simulink model "FSAC2021_V1_Running"  (R2014a)
settings: Solver=FixedStepDiscrete  StartTime=0.0  StopTime=inf  FixedStep=0.0005  RelTol=1e-3
model workspace (MAT data in the model file):
  MCOS : class17 (value not decoded)
  MCOS : class17 (value not decoded)
  MCOS : class17 (value not decoded)
  MCOS : class17 (value not decoded)
  MCOS : class17 (value not decoded)
  MCOS : class17 (value not decoded)
  MCOS : class17 (value not decoded)
  MCOS : class17 (value not decoded)
  MCOS : class17 (value not decoded)
  MCOS : class17 (value not decoded)
  MCOS : class17 (value not decoded)
  MCOS : class17 (value not decoded)
  MCOS : class17 (value not decoded)
  MCOS : class17 (value not decoded)
  MCOS : class17 (value not decoded)
  MCOS : class17 (value not decoded)
  MCOS : class17 (value not decoded)
  MCOS : class17 (value not decoded)
  MCOS : class17 (value not decoded)
  BUZZER_START = 1
  MCOS : class17 (value not decoded)
  MCOS : class17 (value not decoded)
  MCOS : class17 (value not decoded)
  MCOS : class17 (value not decoded)
  MCOS : class17 (value not decoded)
  MCOS : class17 (value not decoded)
  MCOS : class17 (value not decoded)
  MCOS : class17 (value not decoded)
  MCOS : class17 (value not decoded)
  MCOS : class17 (value not decoded)
  MCOS : class17 (value not decoded)
  MCOS : class17 (value not decoded)
  MCOS : class17 (value not decoded)
  MCOS : class17 (value not decoded)
  MCOS : class17 (value not decoded)
  MCOS : class17 (value not decoded)
  MCOS : class17 (value not decoded)
  MCOS : class17 (value not decoded)
  MCOS : class17 (value not decoded)
  MCOS : class17 (value not decoded)
  MCOS : class17 (value not decoded)
  MCOS : class17 (value not decoded)
  MCOS : class17 (value not decoded)
  MCOS : class17 (value not decoded)
  MCOS : class17 (value not decoded)
  MCOS : class17 (value not decoded)
  MCOS : class17 (value not decoded)
  MCOS : class17 (value not decoded)
  MCOS : class17 (value not decoded)
  MCOS : class17 (value not decoded)
  MCOS : class17 (value not decoded)
  MCOS : class17 (value not decoded)
  MCOS : class17 (value not decoded)
  MCOS : class17 (value not decoded)
  MCOS : class17 (value not decoded)
  MCOS : class17 (value not decoded)
  MCOS : class17 (value not decoded)
  MCOS : class17 (value not decoded)
  Brake = 11
  MCOS : class17 (value not decoded)
  MCOS : class17 (value not decoded)
  MCOS : class17 (value not decoded)
  MCOS : class17 (value not decoded)
  MCOS : class17 (value not decoded)
  MCOS : class17 (value not decoded)
  MCOS : class17 (value not decoded)
  MCOS : class17 (value not decoded)
  Sensor_Acc_b = 101.85
  Sensor_Acc_k = -0.0185
  Str_Sen_Orig_Angle = -341
  MCOS : class17 (value not decoded)
  Tire_D = 0.47
  T = 0.05
libraries: simulink x402, ec55xxlib x134
(part 17 of 17)

== system FSAC2021_V1_Running/ROUTING/TO_DCAN/Subsystem/DIAG_VEH_SENSOR/Front_wheel_angle ==
  Front_wheel_angle : Inport
  Constant{1..3,5..8} (7 alike) : Constant  Value=0  OutDataTypeStr=uint8  SampleTime=-1
  Front_wheel_angleABS : Abs
  Front_wheel_angleCS : ArithShift  BitShiftNumber=-8
  Front_wheel_angleConS : Constant  OutDataTypeStr=single
  Front_wheel_angleCosR : Constant  Value=0  OutDataTypeStr=uint8
  Front_wheel_angleROP : RelationalOperator  Operator=<  OutDataTypeStr=boolean
  Front_wheel_angleRon : Rounding  Operator=round
  Front_wheel_angleSW : Switch  Criteria=u2 ~= 0
  Front_wheel_angle_1sat : Saturate  UpperLimit=255  LowerLimit=0
  Front_wheel_angle_Convert : DataTypeConversion  OutDataTypeStr=uint8
  Front_wheel_angle_Convert1 : DataTypeConversion  OutDataTypeStr=uint32
  Front_wheel_angle_D : Product  Inputs=*/
  Front_wheel_angle_F : Constant  OutDataTypeStr=single
  Front_wheel_angle_L : simulink/Logic and Bit Operations/Bitwise Operator  logicop=AND  UseBitMask=on  BitMask=255  BitMaskRealWorld=Stored Integer
  Front_wheel_angle_O : Constant  Value=0  OutDataTypeStr=single
  Front_wheel_angle_S : ArithShift
  Front_wheel_angle_sat : Saturate  UpperLimit=127  LowerLimit=-128
  Front_wheel_angle_st : Sum  Inputs=+-
  Front_wheel_anglesubcon : Sum  Inputs=+-
  output1 : Outport
  output2 : Outport  Port=2
  output3 : Outport  Port=3
  output4 : Outport  Port=4
  output5 : Outport  Port=5
  output6 : Outport  Port=6
  output7 : Outport  Port=7
  output8 : Outport  Port=8
  wires:
  Front_wheel_angle/1 -> Front_wheel_angle_sat/1
  Front_wheel_angle_sat/1 -> Front_wheel_angle_st/1
  Front_wheel_angle_O/1 -> Front_wheel_angle_st/2
  Front_wheel_angle_st/1 -> Front_wheel_angle_D/1
  Front_wheel_angle_F/1 -> Front_wheel_angle_D/2
  Front_wheel_angle_D/1 -> Front_wheel_angleRon/1
  Front_wheel_angleRon/1 -> Front_wheel_angleROP/1, Front_wheel_angleABS/1, Front_wheel_angleSW/3
  Front_wheel_angleCosR/1 -> Front_wheel_angleROP/2
  Front_wheel_angleConS/1 -> Front_wheel_angleCS/1
  Front_wheel_angleCS/1 -> Front_wheel_anglesubcon/1
  Front_wheel_angleABS/1 -> Front_wheel_anglesubcon/2
  Front_wheel_anglesubcon/1 -> Front_wheel_angleSW/1
  Front_wheel_angleROP/1 -> Front_wheel_angleSW/2
  Front_wheel_angleSW/1 -> Front_wheel_angle_S/1
  Front_wheel_angle_S/1 -> Front_wheel_angle_1sat/1
  Front_wheel_angle_1sat/1 -> Front_wheel_angle_Convert1/1
  Front_wheel_angle_Convert1/1 -> Front_wheel_angle_L/1
  Front_wheel_angle_L/1 -> Front_wheel_angle_Convert/1
  Front_wheel_angle_Convert/1 -> output4/1
  Constant1/1 -> output1/1
  Constant2/1 -> output2/1
  Constant3/1 -> output3/1
  Constant5/1 -> output5/1
  Constant6/1 -> output6/1
  Constant7/1 -> output7/1
  Constant8/1 -> output8/1

== system FSAC2021_V1_Running/ROUTING/TO_DCAN/Subsystem/DIAG_VEH_SENSOR/Hydra_Prs ==
  Hydra_Prs : Inport
  Constant{1..4,6..8} (7 alike) : Constant  Value=0  OutDataTypeStr=uint8  SampleTime=-1
  Hydra_PrsRon : Rounding  Operator=round
  Hydra_Prs_1sat : Saturate  UpperLimit=255  LowerLimit=0
  Hydra_Prs_Convert : DataTypeConversion  OutDataTypeStr=uint8
  Hydra_Prs_Convert1 : DataTypeConversion  OutDataTypeStr=uint32
  Hydra_Prs_D : Product  Inputs=*/
  Hydra_Prs_F : Constant  Value=0.1  OutDataTypeStr=single
  Hydra_Prs_L : simulink/Logic and Bit Operations/Bitwise Operator  logicop=AND  UseBitMask=on  BitMask=255  BitMaskRealWorld=Stored Integer
  Hydra_Prs_O : Constant  Value=0  OutDataTypeStr=single
  Hydra_Prs_S : ArithShift
  Hydra_Prs_sat : Saturate  UpperLimit=25.5  LowerLimit=0
  Hydra_Prs_st : Sum  Inputs=+-
  output1 : Outport
  output2 : Outport  Port=2
  output3 : Outport  Port=3
  output4 : Outport  Port=4
  output5 : Outport  Port=5
  output6 : Outport  Port=6
  output7 : Outport  Port=7
  output8 : Outport  Port=8
  wires:
  Hydra_Prs/1 -> Hydra_Prs_sat/1
  Hydra_Prs_sat/1 -> Hydra_Prs_st/1
  Hydra_Prs_O/1 -> Hydra_Prs_st/2
  Hydra_Prs_st/1 -> Hydra_Prs_D/1
  Hydra_Prs_F/1 -> Hydra_Prs_D/2
  Hydra_Prs_D/1 -> Hydra_PrsRon/1
  Hydra_PrsRon/1 -> Hydra_Prs_S/1
  Hydra_Prs_S/1 -> Hydra_Prs_1sat/1
  Hydra_Prs_1sat/1 -> Hydra_Prs_Convert1/1
  Hydra_Prs_Convert1/1 -> Hydra_Prs_L/1
  Hydra_Prs_L/1 -> Hydra_Prs_Convert/1
  Hydra_Prs_Convert/1 -> output5/1
  Constant1/1 -> output1/1
  Constant2/1 -> output2/1
  Constant3/1 -> output3/1
  Constant4/1 -> output4/1
  Constant6/1 -> output6/1
  Constant7/1 -> output7/1
  Constant8/1 -> output8/1

== system FSAC2021_V1_Running/ROUTING/TO_DCAN/Subsystem/DIAG_VEH_SENSOR/Mtr_Input_Volt ==
  Mtr_Input_Volt : Inport
  Constant{1,3..8} (7 alike) : Constant  Value=0  OutDataTypeStr=uint8  SampleTime=-1
  Mtr_Input_VoltRon : Rounding  Operator=round
  Mtr_Input_Volt_1sat : Saturate  UpperLimit=255  LowerLimit=0
  Mtr_Input_Volt_Convert : DataTypeConversion  OutDataTypeStr=uint8
  Mtr_Input_Volt_Convert1 : DataTypeConversion  OutDataTypeStr=uint32
  Mtr_Input_Volt_D : Product  Inputs=*/
  Mtr_Input_Volt_F : Constant  OutDataTypeStr=single
  Mtr_Input_Volt_L : simulink/Logic and Bit Operations/Bitwise Operator  logicop=AND  UseBitMask=on  BitMask=255  BitMaskRealWorld=Stored Integer
  Mtr_Input_Volt_O : Constant  Value=0  OutDataTypeStr=single
  Mtr_Input_Volt_S : ArithShift
  Mtr_Input_Volt_sat : Saturate  UpperLimit=255  LowerLimit=0
  Mtr_Input_Volt_st : Sum  Inputs=+-
  output1 : Outport
  output2 : Outport  Port=2
  output3 : Outport  Port=3
  output4 : Outport  Port=4
  output5 : Outport  Port=5
  output6 : Outport  Port=6
  output7 : Outport  Port=7
  output8 : Outport  Port=8
  wires:
  Mtr_Input_Volt/1 -> Mtr_Input_Volt_sat/1
  Mtr_Input_Volt_sat/1 -> Mtr_Input_Volt_st/1
  Mtr_Input_Volt_O/1 -> Mtr_Input_Volt_st/2
  Mtr_Input_Volt_st/1 -> Mtr_Input_Volt_D/1
  Mtr_Input_Volt_F/1 -> Mtr_Input_Volt_D/2
  Mtr_Input_Volt_D/1 -> Mtr_Input_VoltRon/1
  Mtr_Input_VoltRon/1 -> Mtr_Input_Volt_S/1
  Mtr_Input_Volt_S/1 -> Mtr_Input_Volt_1sat/1
  Mtr_Input_Volt_1sat/1 -> Mtr_Input_Volt_Convert1/1
  Mtr_Input_Volt_Convert1/1 -> Mtr_Input_Volt_L/1
  Mtr_Input_Volt_L/1 -> Mtr_Input_Volt_Convert/1
  Mtr_Input_Volt_Convert/1 -> output2/1
  Constant1/1 -> output1/1
  Constant3/1 -> output3/1
  Constant4/1 -> output4/1
  Constant5/1 -> output5/1
  Constant6/1 -> output6/1
  Constant7/1 -> output7/1
  Constant8/1 -> output8/1

== system FSAC2021_V1_Running/ROUTING/TO_DCAN/Subsystem/DIAG_VEH_SENSOR/Pedal_Acc ==
  Pedal_Acc : Inport
  Constant{1..6} (6 alike) : Constant  Value=0  OutDataTypeStr=uint8  SampleTime=-1
  Pedal_AccBitCov : DataTypeConversion  OutDataTypeStr=uint8
  Pedal_AccCOV : DataTypeConversion  OutDataTypeStr=uint8
  Pedal_AccRon : Rounding  Operator=round
  Pedal_Acc_1sat : Saturate  UpperLimit=16256  LowerLimit=0
  Pedal_Acc_And : simulink/Logic and Bit Operations/Bitwise Operator  logicop=AND  UseBitMask=off  NumInputPorts=2  BitMask=bin2dec('11011001')  BitMaskRealWorld=Stored Integer
  Pedal_Acc_And_C : Constant  Value=255  OutDataTypeStr=uint32
  Pedal_Acc_Convert : DataTypeConversion  OutDataTypeStr=uint32
  Pedal_Acc_D : Product  Inputs=*/
  Pedal_Acc_D1 : Product  Inputs=*/
  Pedal_Acc_F : Constant  OutDataTypeStr=single
  Pedal_Acc_L : simulink/Logic and Bit Operations/Bitwise Operator  logicop=AND  UseBitMask=on  BitMask=16256  BitMaskRealWorld=Stored Integer
  Pedal_Acc_O : Constant  Value=0  OutDataTypeStr=single
  Pedal_Acc_S : ArithShift  BitShiftNumber=-7
  Pedal_Acc_sat : Saturate  UpperLimit=127  LowerLimit=0
  Pedal_Acc_st : Sum  Inputs=+-
  Pedal_Accoutput7_C : Constant  Value=256
  output1 : Outport
  output2 : Outport  Port=2
  output3 : Outport  Port=3
  output4 : Outport  Port=4
  output5 : Outport  Port=5
  output6 : Outport  Port=6
  output7 : Outport  Port=7
  output8 : Outport  Port=8
  wires:
  Pedal_Acc/1 -> Pedal_Acc_sat/1
  Pedal_Acc_sat/1 -> Pedal_Acc_st/1
  Pedal_Acc_O/1 -> Pedal_Acc_st/2
  Pedal_Acc_st/1 -> Pedal_Acc_D/1
  Pedal_Acc_F/1 -> Pedal_Acc_D/2
  Pedal_Acc_D/1 -> Pedal_AccRon/1
  Pedal_AccRon/1 -> Pedal_Acc_S/1
  Pedal_Acc_S/1 -> Pedal_Acc_1sat/1
  Pedal_Acc_1sat/1 -> Pedal_Acc_Convert/1
  Pedal_Acc_Convert/1 -> Pedal_Acc_L/1
  Pedal_Acc_L/1 -> Pedal_Acc_D1/1, Pedal_Acc_And/1
  Pedal_Accoutput7_C/1 -> Pedal_Acc_D1/2
  Pedal_Acc_D1/1 -> Pedal_AccCOV/1
  Pedal_AccCOV/1 -> output7/1
  Pedal_Acc_And_C/1 -> Pedal_Acc_And/2
  Pedal_Acc_And/1 -> Pedal_AccBitCov/1
  Pedal_AccBitCov/1 -> output8/1
  Constant1/1 -> output1/1
  Constant2/1 -> output2/1
  Constant3/1 -> output3/1
  Constant4/1 -> output4/1
  Constant5/1 -> output5/1
  Constant6/1 -> output6/1

== system FSAC2021_V1_Running/ROUTING/TO_DCAN/Subsystem/DIAG_VEH_SENSOR/Pedal_Brake ==
  Pedal_Brake : Inport
  Constant{1..7} (7 alike) : Constant  Value=0  OutDataTypeStr=uint8  SampleTime=-1
  Pedal_BrakeRon : Rounding  Operator=round
  Pedal_Brake_1sat : Saturate  UpperLimit=127  LowerLimit=0
  Pedal_Brake_Convert : DataTypeConversion  OutDataTypeStr=uint8
  Pedal_Brake_Convert1 : DataTypeConversion  OutDataTypeStr=uint32
  Pedal_Brake_D : Product  Inputs=*/
  Pedal_Brake_F : Constant  OutDataTypeStr=single
  Pedal_Brake_L : simulink/Logic and Bit Operations/Bitwise Operator  logicop=AND  UseBitMask=on  BitMask=127  BitMaskRealWorld=Stored Integer
  Pedal_Brake_O : Constant  Value=0  OutDataTypeStr=single
  Pedal_Brake_S : ArithShift
  Pedal_Brake_sat : Saturate  UpperLimit=127  LowerLimit=0
  Pedal_Brake_st : Sum  Inputs=+-
  output1 : Outport
  output2 : Outport  Port=2
  output3 : Outport  Port=3
  output4 : Outport  Port=4
  output5 : Outport  Port=5
  output6 : Outport  Port=6
  output7 : Outport  Port=7
  output8 : Outport  Port=8
  wires:
  Pedal_Brake/1 -> Pedal_Brake_sat/1
  Pedal_Brake_sat/1 -> Pedal_Brake_st/1
  Pedal_Brake_O/1 -> Pedal_Brake_st/2
  Pedal_Brake_st/1 -> Pedal_Brake_D/1
  Pedal_Brake_F/1 -> Pedal_Brake_D/2
  Pedal_Brake_D/1 -> Pedal_BrakeRon/1
  Pedal_BrakeRon/1 -> Pedal_Brake_S/1
  Pedal_Brake_S/1 -> Pedal_Brake_1sat/1
  Pedal_Brake_1sat/1 -> Pedal_Brake_Convert1/1
  Pedal_Brake_Convert1/1 -> Pedal_Brake_L/1
  Pedal_Brake_L/1 -> Pedal_Brake_Convert/1
  Pedal_Brake_Convert/1 -> output8/1
  Constant1/1 -> output1/1
  Constant2/1 -> output2/1
  Constant3/1 -> output3/1
  Constant4/1 -> output4/1
  Constant5/1 -> output5/1
  Constant6/1 -> output6/1
  Constant7/1 -> output7/1

== system FSAC2021_V1_Running/ROUTING/TO_DCAN/Subsystem/DIAG_VEH_SENSOR/Veh_Current_Speed ==
  Veh_Current_Speed : Inport
  Constant{1..5,8} (6 alike) : Constant  Value=0  OutDataTypeStr=uint8  SampleTime=-1
  Veh_Current_SpeedBitCov : DataTypeConversion  OutDataTypeStr=uint8
  Veh_Current_SpeedCOV : DataTypeConversion  OutDataTypeStr=uint8
  Veh_Current_SpeedRon : Rounding  Operator=round
  Veh_Current_Speed_1sat : Saturate  UpperLimit=65472  LowerLimit=0
  Veh_Current_Speed_And : simulink/Logic and Bit Operations/Bitwise Operator  logicop=AND  UseBitMask=off  NumInputPorts=2  BitMask=bin2dec('11011001')  BitMaskRealWorld=Stored Integer
  Veh_Current_Speed_And_C : Constant  Value=255  OutDataTypeStr=uint32
  Veh_Current_Speed_Convert : DataTypeConversion  OutDataTypeStr=uint32
  Veh_Current_Speed_D : Product  Inputs=*/
  Veh_Current_Speed_D1 : Product  Inputs=*/
  Veh_Current_Speed_F : Constant  Value=0.1  OutDataTypeStr=single
  Veh_Current_Speed_L : simulink/Logic and Bit Operations/Bitwise Operator  logicop=AND  UseBitMask=on  BitMask=65472  BitMaskRealWorld=Stored Integer
  Veh_Current_Speed_O : Constant  Value=0  OutDataTypeStr=single
  Veh_Current_Speed_S : ArithShift  BitShiftNumber=-6
  Veh_Current_Speed_sat : Saturate  UpperLimit=102.3  LowerLimit=0
  Veh_Current_Speed_st : Sum  Inputs=+-
  Veh_Current_Speedoutput6_C : Constant  Value=256
  output1 : Outport
  output2 : Outport  Port=2
  output3 : Outport  Port=3
  output4 : Outport  Port=4
  output5 : Outport  Port=5
  output6 : Outport  Port=6
  output7 : Outport  Port=7
  output8 : Outport  Port=8
  wires:
  Veh_Current_Speed/1 -> Veh_Current_Speed_sat/1
  Veh_Current_Speed_sat/1 -> Veh_Current_Speed_st/1
  Veh_Current_Speed_O/1 -> Veh_Current_Speed_st/2
  Veh_Current_Speed_st/1 -> Veh_Current_Speed_D/1
  Veh_Current_Speed_F/1 -> Veh_Current_Speed_D/2
  Veh_Current_Speed_D/1 -> Veh_Current_SpeedRon/1
  Veh_Current_SpeedRon/1 -> Veh_Current_Speed_S/1
  Veh_Current_Speed_S/1 -> Veh_Current_Speed_1sat/1
  Veh_Current_Speed_1sat/1 -> Veh_Current_Speed_Convert/1
  Veh_Current_Speed_Convert/1 -> Veh_Current_Speed_L/1
  Veh_Current_Speed_L/1 -> Veh_Current_Speed_D1/1, Veh_Current_Speed_And/1
  Veh_Current_Speedoutput6_C/1 -> Veh_Current_Speed_D1/2
  Veh_Current_Speed_D1/1 -> Veh_Current_SpeedCOV/1
  Veh_Current_SpeedCOV/1 -> output6/1
  Veh_Current_Speed_And_C/1 -> Veh_Current_Speed_And/2
  Veh_Current_Speed_And/1 -> Veh_Current_SpeedBitCov/1
  Veh_Current_SpeedBitCov/1 -> output7/1
  Constant1/1 -> output1/1
  Constant2/1 -> output2/1
  Constant3/1 -> output3/1
  Constant4/1 -> output4/1
  Constant5/1 -> output5/1
  Constant8/1 -> output8/1

== system FSAC2021_V1_Running/ROUTING/TO_DCAN/Subsystem/DIAG_WHL_SPD/FL_Whl_Spd ==
  FL_Whl_Spd : Inport
  Constant{3..8} (6 alike) : Constant  Value=0  OutDataTypeStr=uint8  SampleTime=-1
  FL_Whl_SpdBitCov : DataTypeConversion  OutDataTypeStr=uint8
  FL_Whl_SpdCOV : DataTypeConversion  OutDataTypeStr=uint8
  FL_Whl_SpdRon : Rounding  Operator=round
  FL_Whl_Spd_1sat : Saturate  UpperLimit=65535  LowerLimit=0
  FL_Whl_Spd_And : simulink/Logic and Bit Operations/Bitwise Operator  logicop=AND  UseBitMask=off  NumInputPorts=2  BitMask=bin2dec('11011001')  BitMaskRealWorld=Stored Integer
  FL_Whl_Spd_And_C : Constant  Value=255  OutDataTypeStr=uint32
  FL_Whl_Spd_Convert : DataTypeConversion  OutDataTypeStr=uint32
  FL_Whl_Spd_D : Product  Inputs=*/
  FL_Whl_Spd_D1 : Product  Inputs=*/
  FL_Whl_Spd_F : Constant  OutDataTypeStr=single
  FL_Whl_Spd_L : simulink/Logic and Bit Operations/Bitwise Operator  logicop=AND  UseBitMask=on  BitMask=65535  BitMaskRealWorld=Stored Integer
  FL_Whl_Spd_O : Constant  Value=0  OutDataTypeStr=single
  FL_Whl_Spd_S : ArithShift
  FL_Whl_Spd_sat : Saturate  UpperLimit=65535  LowerLimit=0
  FL_Whl_Spd_st : Sum  Inputs=+-
  FL_Whl_Spdoutput1_C : Constant  Value=256
  output1 : Outport
  output2 : Outport  Port=2
  output3 : Outport  Port=3
  output4 : Outport  Port=4
  output5 : Outport  Port=5
  output6 : Outport  Port=6
  output7 : Outport  Port=7
  output8 : Outport  Port=8
  wires:
  FL_Whl_Spd/1 -> FL_Whl_Spd_sat/1
  FL_Whl_Spd_sat/1 -> FL_Whl_Spd_st/1
  FL_Whl_Spd_O/1 -> FL_Whl_Spd_st/2
  FL_Whl_Spd_st/1 -> FL_Whl_Spd_D/1
  FL_Whl_Spd_F/1 -> FL_Whl_Spd_D/2
  FL_Whl_Spd_D/1 -> FL_Whl_SpdRon/1
  FL_Whl_SpdRon/1 -> FL_Whl_Spd_S/1
  FL_Whl_Spd_S/1 -> FL_Whl_Spd_1sat/1
  FL_Whl_Spd_1sat/1 -> FL_Whl_Spd_Convert/1
  FL_Whl_Spd_Convert/1 -> FL_Whl_Spd_L/1
  FL_Whl_Spd_L/1 -> FL_Whl_Spd_D1/1, FL_Whl_Spd_And/1
  FL_Whl_Spdoutput1_C/1 -> FL_Whl_Spd_D1/2
  FL_Whl_Spd_D1/1 -> FL_Whl_SpdCOV/1
  FL_Whl_SpdCOV/1 -> output1/1
  FL_Whl_Spd_And_C/1 -> FL_Whl_Spd_And/2
  FL_Whl_Spd_And/1 -> FL_Whl_SpdBitCov/1
  FL_Whl_SpdBitCov/1 -> output2/1
  Constant3/1 -> output3/1
  Constant4/1 -> output4/1
  Constant5/1 -> output5/1
  Constant6/1 -> output6/1
  Constant7/1 -> output7/1
  Constant8/1 -> output8/1

== system FSAC2021_V1_Running/ROUTING/TO_DCAN/Subsystem/DIAG_WHL_SPD/FR_Whl_Spd ==
  FR_Whl_Spd : Inport
  Constant{1..2,5..8} (6 alike) : Constant  Value=0  OutDataTypeStr=uint8  SampleTime=-1
  FR_Whl_SpdBitCov : DataTypeConversion  OutDataTypeStr=uint8
  FR_Whl_SpdCOV : DataTypeConversion  OutDataTypeStr=uint8
  FR_Whl_SpdRon : Rounding  Operator=round
  FR_Whl_Spd_1sat : Saturate  UpperLimit=65535  LowerLimit=0
  FR_Whl_Spd_And : simulink/Logic and Bit Operations/Bitwise Operator  logicop=AND  UseBitMask=off  NumInputPorts=2  BitMask=bin2dec('11011001')  BitMaskRealWorld=Stored Integer
  FR_Whl_Spd_And_C : Constant  Value=255  OutDataTypeStr=uint32
  FR_Whl_Spd_Convert : DataTypeConversion  OutDataTypeStr=uint32
  FR_Whl_Spd_D : Product  Inputs=*/
  FR_Whl_Spd_D1 : Product  Inputs=*/
  FR_Whl_Spd_F : Constant  OutDataTypeStr=single
  FR_Whl_Spd_L : simulink/Logic and Bit Operations/Bitwise Operator  logicop=AND  UseBitMask=on  BitMask=65535  BitMaskRealWorld=Stored Integer
  FR_Whl_Spd_O : Constant  Value=0  OutDataTypeStr=single
  FR_Whl_Spd_S : ArithShift
  FR_Whl_Spd_sat : Saturate  UpperLimit=65535  LowerLimit=0
  FR_Whl_Spd_st : Sum  Inputs=+-
  FR_Whl_Spdoutput3_C : Constant  Value=256
  output1 : Outport
  output2 : Outport  Port=2
  output3 : Outport  Port=3
  output4 : Outport  Port=4
  output5 : Outport  Port=5
  output6 : Outport  Port=6
  output7 : Outport  Port=7
  output8 : Outport  Port=8
  wires:
  FR_Whl_Spd/1 -> FR_Whl_Spd_sat/1
  FR_Whl_Spd_sat/1 -> FR_Whl_Spd_st/1
  FR_Whl_Spd_O/1 -> FR_Whl_Spd_st/2
  FR_Whl_Spd_st/1 -> FR_Whl_Spd_D/1
  FR_Whl_Spd_F/1 -> FR_Whl_Spd_D/2
  FR_Whl_Spd_D/1 -> FR_Whl_SpdRon/1
  FR_Whl_SpdRon/1 -> FR_Whl_Spd_S/1
  FR_Whl_Spd_S/1 -> FR_Whl_Spd_1sat/1
  FR_Whl_Spd_1sat/1 -> FR_Whl_Spd_Convert/1
  FR_Whl_Spd_Convert/1 -> FR_Whl_Spd_L/1
  FR_Whl_Spd_L/1 -> FR_Whl_Spd_D1/1, FR_Whl_Spd_And/1
  FR_Whl_Spdoutput3_C/1 -> FR_Whl_Spd_D1/2
  FR_Whl_Spd_D1/1 -> FR_Whl_SpdCOV/1
  FR_Whl_SpdCOV/1 -> output3/1
  FR_Whl_Spd_And_C/1 -> FR_Whl_Spd_And/2
  FR_Whl_Spd_And/1 -> FR_Whl_SpdBitCov/1
  FR_Whl_SpdBitCov/1 -> output4/1
  Constant1/1 -> output1/1
  Constant2/1 -> output2/1
  Constant5/1 -> output5/1
  Constant6/1 -> output6/1
  Constant7/1 -> output7/1
  Constant8/1 -> output8/1

== system FSAC2021_V1_Running/ROUTING/TO_DCAN/Subsystem/DIAG_WHL_SPD/RL_Whl_Spd ==
  RL_Whl_Spd : Inport
  Constant{1..4,7..8} (6 alike) : Constant  Value=0  OutDataTypeStr=uint8  SampleTime=-1
  RL_Whl_SpdBitCov : DataTypeConversion  OutDataTypeStr=uint8
  RL_Whl_SpdCOV : DataTypeConversion  OutDataTypeStr=uint8
  RL_Whl_SpdRon : Rounding  Operator=round
  RL_Whl_Spd_1sat : Saturate  UpperLimit=65535  LowerLimit=0
  RL_Whl_Spd_And : simulink/Logic and Bit Operations/Bitwise Operator  logicop=AND  UseBitMask=off  NumInputPorts=2  BitMask=bin2dec('11011001')  BitMaskRealWorld=Stored Integer
  RL_Whl_Spd_And_C : Constant  Value=255  OutDataTypeStr=uint32
  RL_Whl_Spd_Convert : DataTypeConversion  OutDataTypeStr=uint32
  RL_Whl_Spd_D : Product  Inputs=*/
  RL_Whl_Spd_D1 : Product  Inputs=*/
  RL_Whl_Spd_F : Constant  OutDataTypeStr=single
  RL_Whl_Spd_L : simulink/Logic and Bit Operations/Bitwise Operator  logicop=AND  UseBitMask=on  BitMask=65535  BitMaskRealWorld=Stored Integer
  RL_Whl_Spd_O : Constant  Value=0  OutDataTypeStr=single
  RL_Whl_Spd_S : ArithShift
  RL_Whl_Spd_sat : Saturate  UpperLimit=65535  LowerLimit=0
  RL_Whl_Spd_st : Sum  Inputs=+-
  RL_Whl_Spdoutput5_C : Constant  Value=256
  output1 : Outport
  output2 : Outport  Port=2
  output3 : Outport  Port=3
  output4 : Outport  Port=4
  output5 : Outport  Port=5
  output6 : Outport  Port=6
  output7 : Outport  Port=7
  output8 : Outport  Port=8
  wires:
  RL_Whl_Spd/1 -> RL_Whl_Spd_sat/1
  RL_Whl_Spd_sat/1 -> RL_Whl_Spd_st/1
  RL_Whl_Spd_O/1 -> RL_Whl_Spd_st/2
  RL_Whl_Spd_st/1 -> RL_Whl_Spd_D/1
  RL_Whl_Spd_F/1 -> RL_Whl_Spd_D/2
  RL_Whl_Spd_D/1 -> RL_Whl_SpdRon/1
  RL_Whl_SpdRon/1 -> RL_Whl_Spd_S/1
  RL_Whl_Spd_S/1 -> RL_Whl_Spd_1sat/1
  RL_Whl_Spd_1sat/1 -> RL_Whl_Spd_Convert/1
  RL_Whl_Spd_Convert/1 -> RL_Whl_Spd_L/1
  RL_Whl_Spd_L/1 -> RL_Whl_Spd_D1/1, RL_Whl_Spd_And/1
  RL_Whl_Spdoutput5_C/1 -> RL_Whl_Spd_D1/2
  RL_Whl_Spd_D1/1 -> RL_Whl_SpdCOV/1
  RL_Whl_SpdCOV/1 -> output5/1
  RL_Whl_Spd_And_C/1 -> RL_Whl_Spd_And/2
  RL_Whl_Spd_And/1 -> RL_Whl_SpdBitCov/1
  RL_Whl_SpdBitCov/1 -> output6/1
  Constant1/1 -> output1/1
  Constant2/1 -> output2/1
  Constant3/1 -> output3/1
  Constant4/1 -> output4/1
  Constant7/1 -> output7/1
  Constant8/1 -> output8/1

== system FSAC2021_V1_Running/ROUTING/TO_DCAN/Subsystem/DIAG_WHL_SPD/RR_Whl_Spd ==
  RR_Whl_Spd : Inport
  Constant{1..6} (6 alike) : Constant  Value=0  OutDataTypeStr=uint8  SampleTime=-1
  RR_Whl_SpdBitCov : DataTypeConversion  OutDataTypeStr=uint8
  RR_Whl_SpdCOV : DataTypeConversion  OutDataTypeStr=uint8
  RR_Whl_SpdRon : Rounding  Operator=round
  RR_Whl_Spd_1sat : Saturate  UpperLimit=65535  LowerLimit=0
  RR_Whl_Spd_And : simulink/Logic and Bit Operations/Bitwise Operator  logicop=AND  UseBitMask=off  NumInputPorts=2  BitMask=bin2dec('11011001')  BitMaskRealWorld=Stored Integer
  RR_Whl_Spd_And_C : Constant  Value=255  OutDataTypeStr=uint32
  RR_Whl_Spd_Convert : DataTypeConversion  OutDataTypeStr=uint32
  RR_Whl_Spd_D : Product  Inputs=*/
  RR_Whl_Spd_D1 : Product  Inputs=*/
  RR_Whl_Spd_F : Constant  OutDataTypeStr=single
  RR_Whl_Spd_L : simulink/Logic and Bit Operations/Bitwise Operator  logicop=AND  UseBitMask=on  BitMask=65535  BitMaskRealWorld=Stored Integer
  RR_Whl_Spd_O : Constant  Value=0  OutDataTypeStr=single
  RR_Whl_Spd_S : ArithShift
  RR_Whl_Spd_sat : Saturate  UpperLimit=65535  LowerLimit=0
  RR_Whl_Spd_st : Sum  Inputs=+-
  RR_Whl_Spdoutput7_C : Constant  Value=256
  output1 : Outport
  output2 : Outport  Port=2
  output3 : Outport  Port=3
  output4 : Outport  Port=4
  output5 : Outport  Port=5
  output6 : Outport  Port=6
  output7 : Outport  Port=7
  output8 : Outport  Port=8
  wires:
  RR_Whl_Spd/1 -> RR_Whl_Spd_sat/1
  RR_Whl_Spd_sat/1 -> RR_Whl_Spd_st/1
  RR_Whl_Spd_O/1 -> RR_Whl_Spd_st/2
  RR_Whl_Spd_st/1 -> RR_Whl_Spd_D/1
  RR_Whl_Spd_F/1 -> RR_Whl_Spd_D/2
  RR_Whl_Spd_D/1 -> RR_Whl_SpdRon/1
  RR_Whl_SpdRon/1 -> RR_Whl_Spd_S/1
  RR_Whl_Spd_S/1 -> RR_Whl_Spd_1sat/1
  RR_Whl_Spd_1sat/1 -> RR_Whl_Spd_Convert/1
  RR_Whl_Spd_Convert/1 -> RR_Whl_Spd_L/1
  RR_Whl_Spd_L/1 -> RR_Whl_Spd_D1/1, RR_Whl_Spd_And/1
  RR_Whl_Spdoutput7_C/1 -> RR_Whl_Spd_D1/2
  RR_Whl_Spd_D1/1 -> RR_Whl_SpdCOV/1
  RR_Whl_SpdCOV/1 -> output7/1
  RR_Whl_Spd_And_C/1 -> RR_Whl_Spd_And/2
  RR_Whl_Spd_And/1 -> RR_Whl_SpdBitCov/1
  RR_Whl_SpdBitCov/1 -> output8/1
  Constant1/1 -> output1/1
  Constant2/1 -> output2/1
  Constant3/1 -> output3/1
  Constant4/1 -> output4/1
  Constant5/1 -> output5/1
  Constant6/1 -> output6/1

== system FSAC2021_V1_Running/VCU_CAN_Read/PCANA(RES、AMI、MOTEC、BRAKE、STEER_SENSOR、IPC)/MOTEC_MOTION /MOTEC_MOTION/Motec_Currt_Ang_Sub ==
  In1 : Inport
  Out1 : Outport
  wires:
  In1/1 -> Out1/1

== system FSAC2021_V1_Running/VCU_CAN_Read/PCANA(RES、AMI、MOTEC、BRAKE、STEER_SENSOR、IPC)/MOTEC_MOTION /MOTEC_MOTION/Motec_Currt_Current_Sub ==
  In1 : Inport
  Out1 : Outport
  wires:
  In1/1 -> Out1/1

== system FSAC2021_V1_Running/VCU_CAN_Read/PCANA(RES、AMI、MOTEC、BRAKE、STEER_SENSOR、IPC)/MOTEC_MOTION /MOTEC_MOTION/Motec_Currt_Position_Sub ==
  In1 : Inport
  Out1 : Outport
  wires:
  In1/1 -> Out1/1

== system FSAC2021_V1_Running/VCU_CAN_Read/PCANA(RES、AMI、MOTEC、BRAKE、STEER_SENSOR、IPC)/Str_Emergency /MOTEC_EMERGENCY/Str_Curr_Error_Fault_Sub ==
  In1 : Inport
  Out1 : Outport
  wires:
  In1/1 -> Out1/1

== system FSAC2021_V1_Running/VCU_CAN_Read/PCANA(RES、AMI、MOTEC、BRAKE、STEER_SENSOR、IPC)/Str_Emergency /MOTEC_EMERGENCY/Str_Encoder_Error_Sub ==
  In1 : Inport
  Out1 : Outport
  wires:
  In1/1 -> Out1/1

== system FSAC2021_V1_Running/VCU_CAN_Read/PCANA(RES、AMI、MOTEC、BRAKE、STEER_SENSOR、IPC)/Str_Emergency /MOTEC_EMERGENCY/Str_Flash_Error_Sub ==
  In1 : Inport
  Out1 : Outport
  wires:
  In1/1 -> Out1/1

== system FSAC2021_V1_Running/VCU_CAN_Read/PCANA(RES、AMI、MOTEC、BRAKE、STEER_SENSOR、IPC)/Str_Emergency /MOTEC_EMERGENCY/Str_I2t_Alarm_Sub ==
  In1 : Inport
  Out1 : Outport
  wires:
  In1/1 -> Out1/1

== system FSAC2021_V1_Running/VCU_CAN_Read/PCANA(RES、AMI、MOTEC、BRAKE、STEER_SENSOR、IPC)/Str_Emergency /MOTEC_EMERGENCY/Str_I2t_Warning_Sub ==
  In1 : Inport
  Out1 : Outport
  wires:
  In1/1 -> Out1/1

== system FSAC2021_V1_Running/VCU_CAN_Read/PCANA(RES、AMI、MOTEC、BRAKE、STEER_SENSOR、IPC)/Str_Emergency /MOTEC_EMERGENCY/Str_Limit_Pos_Alarm_Sub ==
  In1 : Inport
  Out1 : Outport
  wires:
  In1/1 -> Out1/1

== system FSAC2021_V1_Running/VCU_CAN_Read/PCANA(RES、AMI、MOTEC、BRAKE、STEER_SENSOR、IPC)/Str_Emergency /MOTEC_EMERGENCY/Str_Over_PosError_Sub ==
  In1 : Inport
  Out1 : Outport
  wires:
  In1/1 -> Out1/1

== system FSAC2021_V1_Running/VCU_CAN_Read/PCANA(RES、AMI、MOTEC、BRAKE、STEER_SENSOR、IPC)/Str_Emergency /MOTEC_EMERGENCY/Str_Over_SpdError_Sub ==
  In1 : Inport
  Out1 : Outport
  wires:
  In1/1 -> Out1/1

== system FSAC2021_V1_Running/VCU_CAN_Read/PCANA(RES、AMI、MOTEC、BRAKE、STEER_SENSOR、IPC)/Str_Emergency /MOTEC_EMERGENCY/Str_Over_TopCurr_Sub ==
  In1 : Inport
  Out1 : Outport
  wires:
  In1/1 -> Out1/1

== system FSAC2021_V1_Running/VCU_CAN_Read/PCANA(RES、AMI、MOTEC、BRAKE、STEER_SENSOR、IPC)/Str_Emergency /MOTEC_EMERGENCY/Str_Overvolt_Warning_Sub ==
  In1 : Inport
  Out1 : Outport
  wires:
  In1/1 -> Out1/1

== system FSAC2021_V1_Running/VCU_CAN_Read/PCANA(RES、AMI、MOTEC、BRAKE、STEER_SENSOR、IPC)/Str_Emergency /MOTEC_EMERGENCY/Str_Para_Error_Sub ==
  In1 : Inport
  Out1 : Outport
  wires:
  In1/1 -> Out1/1

== system FSAC2021_V1_Running/VCU_CAN_Read/PCANA(RES、AMI、MOTEC、BRAKE、STEER_SENSOR、IPC)/Str_Emergency /MOTEC_EMERGENCY/Str_PwrMod_TempHigh_Alarm_Sub ==
  In1 : Inport
  Out1 : Outport
  wires:
  In1/1 -> Out1/1

== system FSAC2021_V1_Running/VCU_CAN_Read/PCANA(RES、AMI、MOTEC、BRAKE、STEER_SENSOR、IPC)/Str_Emergency /MOTEC_EMERGENCY/Str_PwrMod_TempHigh_Warning_Sub ==
  In1 : Inport
  Out1 : Outport
  wires:
  In1/1 -> Out1/1

== system FSAC2021_V1_Running/VCU_CAN_Read/PCANA(RES、AMI、MOTEC、BRAKE、STEER_SENSOR、IPC)/Str_Emergency /MOTEC_EMERGENCY/Str_Spd_Over_Alam_Sub ==
  In1 : Inport
  Out1 : Outport
  wires:
  In1/1 -> Out1/1

== system FSAC2021_V1_Running/VCU_CAN_Read/PCANA(RES、AMI、MOTEC、BRAKE、STEER_SENSOR、IPC)/Str_Emergency /MOTEC_EMERGENCY/Str_System_Error_Sub ==
  In1 : Inport
  Out1 : Outport
  wires:
  In1/1 -> Out1/1

== system FSAC2021_V1_Running/VCU_CAN_Read/PCANA(RES、AMI、MOTEC、BRAKE、STEER_SENSOR、IPC)/Str_Emergency /MOTEC_EMERGENCY/Str_UnderVolt_Warning_Sub ==
  In1 : Inport
  Out1 : Outport
  wires:
  In1/1 -> Out1/1

== system FSAC2021_V1_Running/VCU_CAN_Read/PCANB(BMS、DRIVE_MOTOR)/BMS_ALARM /BMS_HCU_ALARM/ALM_AUX_FAIL_Sub ==
  In1 : Inport
  Out1 : Outport
  wires:
  In1/1 -> Out1/1

== system FSAC2021_V1_Running/VCU_CAN_Read/PCANB(BMS、DRIVE_MOTOR)/BMS_ALARM /BMS_HCU_ALARM/ALM_BATT_DT_Sub ==
  In1 : Inport
  Out1 : Outport
  wires:
  In1/1 -> Out1/1

== system FSAC2021_V1_Running/VCU_CAN_Read/PCANB(BMS、DRIVE_MOTOR)/BMS_ALARM /BMS_HCU_ALARM/ALM_BATT_DV_Sub ==
  In1 : Inport
  Out1 : Outport
  wires:
  In1/1 -> Out1/1

== system FSAC2021_V1_Running/VCU_CAN_Read/PCANB(BMS、DRIVE_MOTOR)/BMS_ALARM /BMS_HCU_ALARM/ALM_BATT_OC_Sub ==
  In1 : Inport
  Out1 : Outport
  wires:
  In1/1 -> Out1/1

== system FSAC2021_V1_Running/VCU_CAN_Read/PCANB(BMS、DRIVE_MOTOR)/BMS_ALARM /BMS_HCU_ALARM/ALM_BATT_OV_Sub ==
  In1 : Inport
  Out1 : Outport
  wires:
  In1/1 -> Out1/1

== system FSAC2021_V1_Running/VCU_CAN_Read/PCANB(BMS、DRIVE_MOTOR)/BMS_ALARM /BMS_HCU_ALARM/ALM_BATT_UC_Sub ==
  In1 : Inport
  Out1 : Outport
  wires:
  In1/1 -> Out1/1

== system FSAC2021_V1_Running/VCU_CAN_Read/PCANB(BMS、DRIVE_MOTOR)/BMS_ALARM /BMS_HCU_ALARM/ALM_BATT_UV_Sub ==
  In1 : Inport
  Out1 : Outport
  wires:
  In1/1 -> Out1/1

== system FSAC2021_V1_Running/VCU_CAN_Read/PCANB(BMS、DRIVE_MOTOR)/BMS_ALARM /BMS_HCU_ALARM/ALM_BMU_FAIL_Sub ==
  In1 : Inport
  Out1 : Outport
  wires:
  In1/1 -> Out1/1

== system FSAC2021_V1_Running/VCU_CAN_Read/PCANB(BMS、DRIVE_MOTOR)/BMS_ALARM /BMS_HCU_ALARM/ALM_BSU_FAULT_Sub ==
  In1 : Inport
  Out1 : Outport
  wires:
  In1/1 -> Out1/1

== system FSAC2021_V1_Running/VCU_CAN_Read/PCANB(BMS、DRIVE_MOTOR)/BMS_ALARM /BMS_HCU_ALARM/ALM_BSU_OFFLINE_Sub ==
  In1 : Inport
  Out1 : Outport
  wires:
  In1/1 -> Out1/1

== system FSAC2021_V1_Running/VCU_CAN_Read/PCANB(BMS、DRIVE_MOTOR)/BMS_ALARM /BMS_HCU_ALARM/ALM_CELL_IBK_Sub ==
  In1 : Inport
  Out1 : Outport
  wires:
  In1/1 -> Out1/1

== system FSAC2021_V1_Running/VCU_CAN_Read/PCANB(BMS、DRIVE_MOTOR)/BMS_ALARM /BMS_HCU_ALARM/ALM_CELL_OT_Sub ==
  In1 : Inport
  Out1 : Outport
  wires:
  In1/1 -> Out1/1

== system FSAC2021_V1_Running/VCU_CAN_Read/PCANB(BMS、DRIVE_MOTOR)/BMS_ALARM /BMS_HCU_ALARM/ALM_CELL_OV_Sub ==
  In1 : Inport
  Out1 : Outport
  wires:
  In1/1 -> Out1/1

== system FSAC2021_V1_Running/VCU_CAN_Read/PCANB(BMS、DRIVE_MOTOR)/BMS_ALARM /BMS_HCU_ALARM/ALM_CELL_TBK_Sub ==
  In1 : Inport
  Out1 : Outport
  wires:
  In1/1 -> Out1/1

== system FSAC2021_V1_Running/VCU_CAN_Read/PCANB(BMS、DRIVE_MOTOR)/BMS_ALARM /BMS_HCU_ALARM/ALM_CELL_UT_Sub ==
  In1 : Inport
  Out1 : Outport
  wires:
  In1/1 -> Out1/1

== system FSAC2021_V1_Running/VCU_CAN_Read/PCANB(BMS、DRIVE_MOTOR)/BMS_ALARM /BMS_HCU_ALARM/ALM_CELL_UV_Sub ==
  In1 : Inport
  Out1 : Outport
  wires:
  In1/1 -> Out1/1

== system FSAC2021_V1_Running/VCU_CAN_Read/PCANB(BMS、DRIVE_MOTOR)/BMS_ALARM /BMS_HCU_ALARM/ALM_CHRG_OCS_Sub ==
  In1 : Inport
  Out1 : Outport
  wires:
  In1/1 -> Out1/1

== system FSAC2021_V1_Running/VCU_CAN_Read/PCANB(BMS、DRIVE_MOTOR)/BMS_ALARM /BMS_HCU_ALARM/ALM_CHRG_OCT_Sub ==
  In1 : Inport
  Out1 : Outport
  wires:
  In1/1 -> Out1/1

== system FSAC2021_V1_Running/VCU_CAN_Read/PCANB(BMS、DRIVE_MOTOR)/BMS_ALARM /BMS_HCU_ALARM/ALM_DSCH_OCS_Sub ==
  In1 : Inport
  Out1 : Outport
  wires:
  In1/1 -> Out1/1

== system FSAC2021_V1_Running/VCU_CAN_Read/PCANB(BMS、DRIVE_MOTOR)/BMS_ALARM /BMS_HCU_ALARM/ALM_DSCH_OCT_Sub ==
  In1 : Inport
  Out1 : Outport
  wires:
  In1/1 -> Out1/1

== system FSAC2021_V1_Running/VCU_CAN_Read/PCANB(BMS、DRIVE_MOTOR)/BMS_ALARM /BMS_HCU_ALARM/ALM_HALL_BREAK_Sub ==
  In1 : Inport
  Out1 : Outport
  wires:
  In1/1 -> Out1/1

== system FSAC2021_V1_Running/VCU_CAN_Read/PCANB(BMS、DRIVE_MOTOR)/BMS_ALARM /BMS_HCU_ALARM/ALM_HVREL_FAIL_Sub ==
  In1 : Inport
  Out1 : Outport
  wires:
  In1/1 -> Out1/1

== system FSAC2021_V1_Running/VCU_CAN_Read/PCANB(BMS、DRIVE_MOTOR)/BMS_ALARM /BMS_HCU_ALARM/ALM_LEAK_OC_Sub ==
  In1 : Inport
  Out1 : Outport
  wires:
  In1/1 -> Out1/1

== system FSAC2021_V1_Running/VCU_CAN_Read/PCANB(BMS、DRIVE_MOTOR)/BMS_ALARM /BMS_HCU_ALARM/ALM_PRECHRG_FAIL_Sub ==
  In1 : Inport
  Out1 : Outport
  wires:
  In1/1 -> Out1/1

== system FSAC2021_V1_Running/VCU_CAN_Read/PCANB(BMS、DRIVE_MOTOR)/BMS_ALARM /BMS_HCU_ALARM/ALM_VCU_OFFLINE_Sub ==
  In1 : Inport
  Out1 : Outport
  wires:
  In1/1 -> Out1/1

== system FSAC2021_V1_Running/VCU_CAN_Read/PCANB(BMS、DRIVE_MOTOR)/BMS_HCU_MAXV /BMS_HCU_MAXV/MaxCellVoltNo_Sub ==
  In1 : Inport
  Out1 : Outport
  wires:
  In1/1 -> Out1/1

== system FSAC2021_V1_Running/VCU_CAN_Read/PCANB(BMS、DRIVE_MOTOR)/BMS_HCU_MAXV /BMS_HCU_MAXV/MaxCellVolt_Sub ==
  In1 : Inport
  Out1 : Outport
  wires:
  In1/1 -> Out1/1

== system FSAC2021_V1_Running/VCU_CAN_Read/PCANB(BMS、DRIVE_MOTOR)/BMS_HCU_MAXV /BMS_HCU_MAXV/MinCellVoltNo_Sub ==
  In1 : Inport
  Out1 : Outport
  wires:
  In1/1 -> Out1/1

== system FSAC2021_V1_Running/VCU_CAN_Read/PCANB(BMS、DRIVE_MOTOR)/BMS_HCU_MAXV /BMS_HCU_MAXV/MinCellVolt_Sub ==
  In1 : Inport
  Out1 : Outport
  wires:
  In1/1 -> Out1/1

== system FSAC2021_V1_Running/VCU_CAN_Read/PCANB(BMS、DRIVE_MOTOR)/BMS_HCU_POWER /BMS_HCU_POWER/MaxChrCurtLimit_Sub ==
  In1 : Inport
  Out1 : Outport
  wires:
  In1/1 -> Out1/1

== system FSAC2021_V1_Running/VCU_CAN_Read/PCANB(BMS、DRIVE_MOTOR)/BMS_HCU_POWER /BMS_HCU_POWER/MaxChrPowerLimit_Sub ==
  In1 : Inport
  Out1 : Outport
  wires:
  In1/1 -> Out1/1

== system FSAC2021_V1_Running/VCU_CAN_Read/PCANB(BMS、DRIVE_MOTOR)/BMS_HCU_POWER /BMS_HCU_POWER/MaxDisCurtLimit_Sub ==
  In1 : Inport
  Out1 : Outport
  wires:
  In1/1 -> Out1/1

== system FSAC2021_V1_Running/VCU_CAN_Read/PCANB(BMS、DRIVE_MOTOR)/BMS_HCU_POWER /BMS_HCU_POWER/MaxDisPowerLimit_Sub ==
  In1 : Inport
  Out1 : Outport
  wires:
  In1/1 -> Out1/1

== system FSAC2021_V1_Running/VCU_CAN_Read/PCANB(BMS、DRIVE_MOTOR)/BMS_RELAY /BMS_HCU_RELAY/ChrCommunication_Sub ==
  In1 : Inport
  Out1 : Outport
  wires:
  In1/1 -> Out1/1

== system FSAC2021_V1_Running/VCU_CAN_Read/PCANB(BMS、DRIVE_MOTOR)/BMS_RELAY /BMS_HCU_RELAY/ChrReqCurr_Sub ==
  In1 : Inport
  Out1 : Outport
  wires:
  In1/1 -> Out1/1

== system FSAC2021_V1_Running/VCU_CAN_Read/PCANB(BMS、DRIVE_MOTOR)/BMS_RELAY /BMS_HCU_RELAY/ChrReqVolt_Sub ==
  In1 : Inport
  Out1 : Outport
  wires:
  In1/1 -> Out1/1

== system FSAC2021_V1_Running/VCU_CAN_Read/PCANB(BMS、DRIVE_MOTOR)/BMS_RELAY /BMS_HCU_RELAY/ChrState_Sub ==
  In1 : Inport
  Out1 : Outport
  wires:
  In1/1 -> Out1/1

== system FSAC2021_V1_Running/VCU_CAN_Read/PCANB(BMS、DRIVE_MOTOR)/BMS_RELAY /BMS_HCU_RELAY/NegRlyStr_Sub ==
  In1 : Inport
  Out1 : Outport
  wires:
  In1/1 -> Out1/1

== system FSAC2021_V1_Running/VCU_CAN_Read/PCANB(BMS、DRIVE_MOTOR)/BMS_RELAY /BMS_HCU_RELAY/OnChrRlyStr_Sub ==
  In1 : Inport
  Out1 : Outport
  wires:
  In1/1 -> Out1/1

== system FSAC2021_V1_Running/VCU_CAN_Read/PCANB(BMS、DRIVE_MOTOR)/BMS_RELAY /BMS_HCU_RELAY/PosRlyStr_Sub ==
  In1 : Inport
  Out1 : Outport
  wires:
  In1/1 -> Out1/1

== system FSAC2021_V1_Running/VCU_CAN_Read/PCANB(BMS、DRIVE_MOTOR)/BMS_RELAY /BMS_HCU_RELAY/PreRlyStr_Sub ==
  In1 : Inport
  Out1 : Outport
  wires:
  In1/1 -> Out1/1

== system FSAC2021_V1_Running/VCU_CAN_Read/PCANB(BMS、DRIVE_MOTOR)/BMS_RELAY /BMS_HCU_RELAY/chrOFFCC2_Sub ==
  In1 : Inport
  Out1 : Outport
  wires:
  In1/1 -> Out1/1

== system FSAC2021_V1_Running/VCU_CAN_Read/PCANB(BMS、DRIVE_MOTOR)/BMS_RELAY /BMS_HCU_RELAY/chrONCC_Sub ==
  In1 : Inport
  Out1 : Outport
  wires:
  In1/1 -> Out1/1

== system FSAC2021_V1_Running/VCU_CAN_Read/PCANB(BMS、DRIVE_MOTOR)/BMS_RELAY /BMS_HCU_RELAY/offChrRlyStr_Sub ==
  In1 : Inport
  Out1 : Outport
  wires:
  In1/1 -> Out1/1

== system FSAC2021_V1_Running/VCU_CAN_Read/Subsystem/BMS_HCU_INFO /BMS_HCU_INFO/BatAlmLv_Sub ==
  In1 : Inport
  Out1 : Outport
  wires:
  In1/1 -> Out1/1

== system FSAC2021_V1_Running/VCU_CAN_Read/Subsystem/BMS_HCU_INFO /BMS_HCU_INFO/BatCurrent_Sub ==
  In1 : Inport
  Out1 : Outport
  wires:
  In1/1 -> Out1/1

== system FSAC2021_V1_Running/VCU_CAN_Read/Subsystem/BMS_HCU_INFO /BMS_HCU_INFO/BatLife_Sub ==
  In1 : Inport
  Out1 : Outport
  wires:
  In1/1 -> Out1/1

== system FSAC2021_V1_Running/VCU_CAN_Read/Subsystem/BMS_HCU_INFO /BMS_HCU_INFO/BatSoc_Sub ==
  In1 : Inport
  Out1 : Outport
  wires:
  In1/1 -> Out1/1

== system FSAC2021_V1_Running/VCU_CAN_Read/Subsystem/BMS_HCU_INFO /BMS_HCU_INFO/BatSoh_Sub ==
  In1 : Inport
  Out1 : Outport
  wires:
  In1/1 -> Out1/1

== system FSAC2021_V1_Running/VCU_CAN_Read/Subsystem/BMS_HCU_INFO /BMS_HCU_INFO/BatState_Sub ==
  In1 : Inport
  Out1 : Outport
  wires:
  In1/1 -> Out1/1

== system FSAC2021_V1_Running/VCU_CAN_Read/Subsystem/BMS_HCU_INFO /BMS_HCU_INFO/BatVoltage_Sub ==
  In1 : Inport
  Out1 : Outport
  wires:
  In1/1 -> Out1/1

== system FSAC2021_V1_Running/VCU_CAN_Read/Subsystem1/HEARTBEAT /MOTEC_HEARTBEAT/Heartbeat_info_Sub ==
  In1 : Inport
  Out1 : Outport
  wires:
  In1/1 -> Out1/1

== system FSAC2021_V1_Running/VCU_CAN_Read/Subsystem2/MOTEC_STATUS /MOTEC_STATUS/Fault_Sub ==
  In1 : Inport
  Out1 : Outport
  wires:
  In1/1 -> Out1/1

== system FSAC2021_V1_Running/VCU_CAN_Read/Subsystem2/MOTEC_STATUS /MOTEC_STATUS/Operation_Enabled_Sub ==
  In1 : Inport
  Out1 : Outport
  wires:
  In1/1 -> Out1/1

== system FSAC2021_V1_Running/VCU_CAN_Read/Subsystem2/MOTEC_STATUS /MOTEC_STATUS/Quick_Stop_Sub ==
  In1 : Inport
  Out1 : Outport
  wires:
  In1/1 -> Out1/1

== system FSAC2021_V1_Running/VCU_CAN_Read/Subsystem2/MOTEC_STATUS /MOTEC_STATUS/Ready_Switch_On_Sub ==
  In1 : Inport
  Out1 : Outport
  wires:
  In1/1 -> Out1/1

== system FSAC2021_V1_Running/VCU_CAN_Read/Subsystem2/MOTEC_STATUS /MOTEC_STATUS/Switch_On_Disabled_Sub ==
  In1 : Inport
  Out1 : Outport
  wires:
  In1/1 -> Out1/1

== system FSAC2021_V1_Running/VCU_CAN_Read/Subsystem2/MOTEC_STATUS /MOTEC_STATUS/Swtiched_On_Sub ==
  In1 : Inport
  Out1 : Outport
  wires:
  In1/1 -> Out1/1

== system FSAC2021_V1_Running/VCU_CAN_Read/Subsystem2/MOTEC_STATUS /MOTEC_STATUS/Target_Reached_Sub ==
  In1 : Inport
  Out1 : Outport
  wires:
  In1/1 -> Out1/1

== system FSAC2021_V1_Running/VCU_CAN_Read/Subsystem2/MOTEC_STATUS /MOTEC_STATUS/Voltage_Enabled_Sub ==
  In1 : Inport
  Out1 : Outport
  wires:
  In1/1 -> Out1/1

== system FSAC2021_V1_Running/VCU_CAN_Read/Subsystem2/MOTEC_STATUS /MOTEC_STATUS/Warning_Sub ==
  In1 : Inport
  Out1 : Outport
  wires:
  In1/1 -> Out1/1
